simulink model "SH_model3"  (R2022b)
settings: Solver=VariableStepAuto  StartTime=0.0  StopTime=10  RelTol=1e-3
InitFcn:
  | f = 50;
  | V = 12;
  | L = 2.8*10^(-3);
  | I_lim = 1.7;
  | psi = L*I_lim;
  | step_angle = 1.8;
  | m = 2;
  | p = 360/(2*step_angle*m);
  | Jr = 5.4*10^(-6);
  | Ra = 1.5;
  | Rb = Ra;
  | Mst = 0.022;
  | B = 3*10^(-3);
  | Mn = 0.004;
  | n = 2;
  | k = 2;
  | q = 0.005;
  | STEP = 1;
  | DIR = 1;
  | microsteps = 1;
  | ENABLE = 1;
undefined symbols (not defined in the file): sigbuilder_block
settings Model: Creator=longp  LastModifiedBy=longp

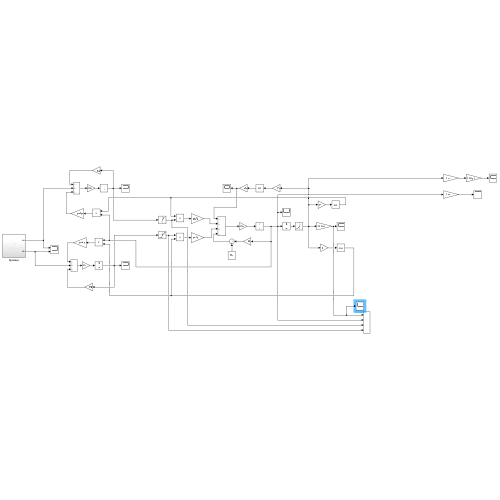
[thumbnail: Simulink's stored preview of the top-level diagram]
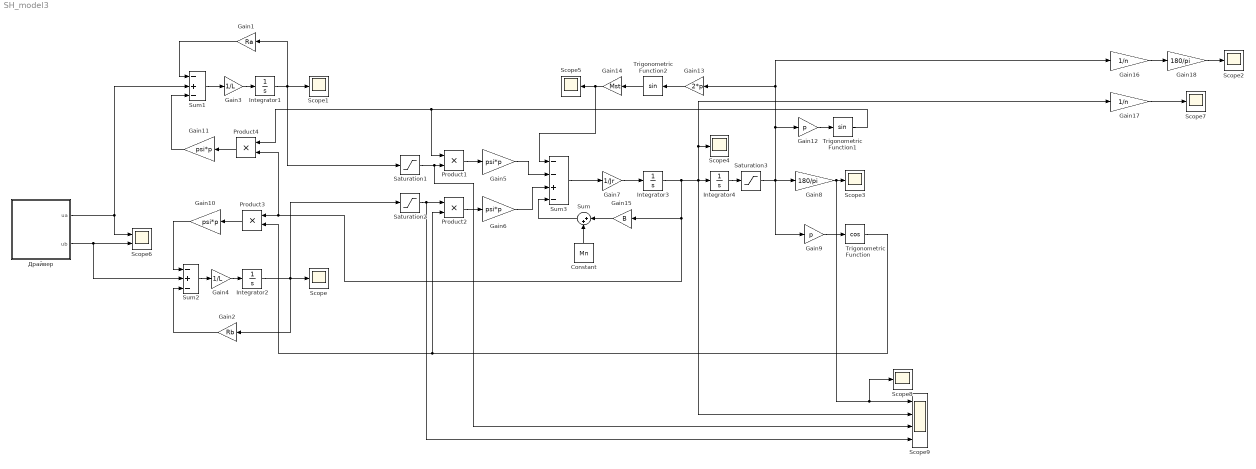
== system SH_model3 ==
  Constant : Constant  Value=Mn
  Gain1 : Gain  Gain=Ra
  Gain{5..6,10..11} (4 alike) : Gain  Gain=psi*p
  Gain12 : Gain  Gain=p
  Gain13 : Gain  Gain=2*p
  Gain14 : Gain  Gain=Mst
  Gain15 : Gain  Gain=B
  Gain16 : Gain  Gain=1/n
  Gain17 : Gain  Gain=1/n
  Gain18 : Gain  Gain=180/pi
  Gain2 : Gain  Gain=Rb
  Gain3 : Gain  Gain=1/L
  Gain4 : Gain  Gain=1/L
  Gain7 : Gain  Gain=1/Jr
  Gain8 : Gain  Gain=180/pi
  Gain9 : Gain  Gain=p
  Integrator{1..4} (4 alike) : Integrator
  Product{1..4} (4 alike) : Product
  Saturation1 : Saturate  UpperLimit=I_lim  LowerLimit=-I_lim
  Saturation2 : Saturate  UpperLimit=I_lim  LowerLimit=-I_lim  ZeroCross=off
  Saturation3 : Saturate  UpperLimit=2*pi  LowerLimit=-2*pi
  Scope{,1..5,7..8} (8 alike) : Scope
  Scope6 : Scope  NumInputPorts=2
  Scope9 : Scope  NumInputPorts=4
  Sum : Sum  Inputs=|++
  Sum1 : Sum  Inputs=-+-
  Sum2 : Sum  Inputs=-+-
  Sum3 : Sum  Inputs=--+-
  Trigonometric Function : Trigonometry  Operator=cos
  Trigonometric Function1 : Trigonometry
  Trigonometric Function2 : Trigonometry
  Драйвер : Subsystem
  wires:
  Integrator1/1 -> Saturation1/1, Gain1/1, Scope1/1
  Gain1/1 -> Sum1/1
  Sum1/1 -> Gain3/1
  Sum2/1 -> Gain4/1
  Integrator2/1 -> Saturation2/1, Gain2/1, Scope/1
  Gain3/1 -> Integrator1/1
  Gain2/1 -> Sum2/3
  Gain4/1 -> Integrator2/1
  Saturation1/1 -> Scope9/3, Product1/2
  Saturation2/1 -> Scope9/4, Product2/1
  Product1/1 -> Gain5/1
  Product2/1 -> Gain6/1
  Gain5/1 -> Sum3/2
  Gain6/1 -> Sum3/3
  Gain7/1 -> Integrator3/1
  Sum3/1 -> Gain7/1
  Integrator4/1 -> Saturation3/1
  Gain9/1 -> Trigonometric Function/1
  Product3/1 -> Gain10/1
  Gain10/1 -> Sum2/1
  Trigonometric Function/1 -> Product2/2, Product3/2
  Product4/1 -> Gain11/1
  Gain11/1 -> Sum1/3
  Gain12/1 -> Trigonometric Function1/1
  Trigonometric Function1/1 -> Product1/1, Product4/1
  Gain13/1 -> Trigonometric Function2/1
  Trigonometric Function2/1 -> Gain14/1
  Gain14/1 -> Sum3/1, Scope5/1
  Integrator3/1 -> Scope9/2, Gain17/1, Scope4/1, Integrator4/1, Product4/2, Product3/1, Gain15/1
  Драйвер/2(ub) -> Sum2/2, Scope6/2
  Драйвер/1(ua) -> Sum1/2, Scope6/1
  Gain8/1 -> Scope8/1, Scope9/1, Scope3/1
  Saturation3/1 -> Gain16/1, Gain13/1, Gain12/1, Gain9/1, Gain8/1
  Constant/1 -> Sum/2
  Gain15/1 -> Sum/1
  Sum/1 -> Sum3/4
  Gain16/1 -> Gain18/1
  Gain17/1 -> Scope7/1
  Gain18/1 -> Scope2/1

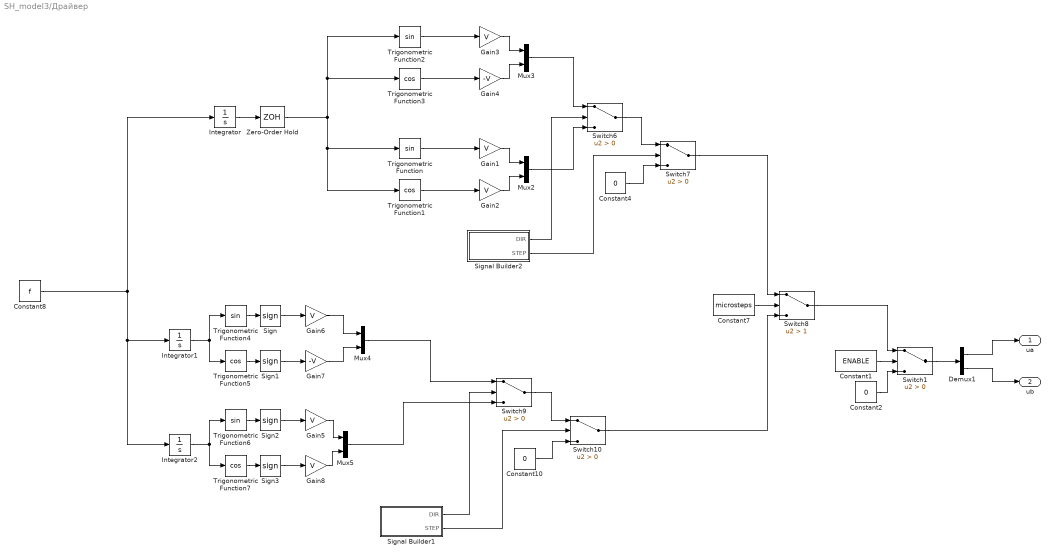
== system SH_model3/Драйвер ==
  Constant1 : Constant  Value=ENABLE
  Constant10 : Constant  Value=0
  Constant2 : Constant  Value=0
  Constant4 : Constant  Value=0
  Constant7 : Constant  Value=microsteps
  Constant8 : Constant  Value=f
  Demux1 : Demux  Outputs=2
  Gain{1..3,5..6,8} (6 alike) : Gain  Gain=V
  Gain4 : Gain  Gain=-V
  Gain7 : Gain  Gain=-V
  Integrator : Integrator
  Integrator1 : Integrator
  Integrator2 : Integrator
  Mux{2..5} (4 alike) : Mux  Inputs=2
  Sign{,1..3} (4 alike) : Signum
  Signal Builder1 : Subsystem  Tag=STV Subsys  LoadFcn=sigbuilder_block('load');  StartFcn=sigbuilder_block('start');  StopFcn=sigbuilder_block('stop');  ClipboardFcn=sigbuilder_block('clipboard');  mask(Sigbuilder block){tuvar=[0:10]}
      mask help: Simulink:masks:SigbuilderBlock_MD
      mask init:
      | if ~strcmp(get_param(bdroot(gcbh),'SimulationStatus'),'stopped') tuvar = sigbuilder_block('maskInit'); end
      settings: CopyFcn=sigbuilder_block('copy');  DeleteFcn=sigbuilder_block('delete');  ModelCloseFcn=sigbuilder_block('modelClose');  PreSaveFcn=sigbuilder_block('preSave');  PauseFcn=sigbuilder_block('pause');  ContinueFcn=sigbuilder_block('continue');  NameChangeFcn=sigbuilder_block('namechange');  OpenFcn=sigbuilder_block('open',[437.6 199.2 550.4 400 ]);  CloseFcn=sigbuilder_block('close');
      mask Display: plot(0, 0, 100, 100,[2, 2, 32, 32, 2], [68, 8, 8, 68, 68],[32, 2], [38, 38], [32, 19, 2],[53, 60, 44], [32, 17, 17, 2],[16, 16, 31, 31]);txt = getActiveGroup(gcbh);text(2, 100, txt,'verticalAlignment', 'top');
  Signal Builder2 : Subsystem  Tag=STV Subsys  LoadFcn=sigbuilder_block('load');  StartFcn=sigbuilder_block('start');  StopFcn=sigbuilder_block('stop');  ClipboardFcn=sigbuilder_block('clipboard');  mask(Sigbuilder block){tuvar=[0:10]}
      mask help: Simulink:masks:SigbuilderBlock_MD
      mask init:
      | if ~strcmp(get_param(bdroot(gcbh),'SimulationStatus'),'stopped') tuvar = sigbuilder_block('maskInit'); end
      settings: CopyFcn=sigbuilder_block('copy');  DeleteFcn=sigbuilder_block('delete');  ModelCloseFcn=sigbuilder_block('modelClose');  PreSaveFcn=sigbuilder_block('preSave');  PauseFcn=sigbuilder_block('pause');  ContinueFcn=sigbuilder_block('continue');  NameChangeFcn=sigbuilder_block('namechange');  OpenFcn=sigbuilder_block('open',[437.6 199.2 550.4 400 ]);  CloseFcn=sigbuilder_block('close');
      mask Display: plot(0, 0, 100, 100,[2, 2, 32, 32, 2], [68, 8, 8, 68, 68],[32, 2], [38, 38], [32, 19, 2],[53, 60, 44], [32, 17, 17, 2],[16, 16, 31, 31]);txt = getActiveGroup(gcbh);text(2, 100, txt,'verticalAlignment', 'top');
  Switch{1,6..7,9..10} (5 alike) : Switch  Criteria=u2 > Threshold  SaturateOnIntegerOverflow=off  InputSameDT=off
  Switch8 : Switch  Criteria=u2 > Threshold  Threshold=1  SaturateOnIntegerOverflow=off  InputSameDT=off
  Trigonometric Function{,2,4,6} (4 alike) : Trigonometry
  Trigonometric Function{1,3,5,7} (4 alike) : Trigonometry  Operator=cos
  Zero-Order Hold : ZeroOrderHold  SampleTime=(2*pi/f)/(2*microsteps)
  ua : Outport
  ub : Outport  Port=2
  wires:
  Switch6/1 -> Switch7/1
  Constant4/1 -> Switch7/3
  Gain2/1 -> Mux2/2
  Gain1/1 -> Mux2/1
  Mux2/1 -> Switch6/3
  Gain4/1 -> Mux3/2
  Gain3/1 -> Mux3/1
  Mux3/1 -> Switch6/1
  Signal Builder2/2(STEP) -> Switch7/2
  Signal Builder2/1(DIR) -> Switch6/2
  Trigonometric Function2/1 -> Gain3/1
  Trigonometric Function3/1 -> Gain4/1
  Trigonometric Function/1 -> Gain1/1
  Trigonometric Function1/1 -> Gain2/1
  Integrator/1 -> Zero-Order Hold/1
  Zero-Order Hold/1 -> Trigonometric Function1/1, Trigonometric Function/1, Trigonometric Function3/1, Trigonometric Function2/1
  Constant7/1 -> Switch8/2
  Integrator1/1 -> Trigonometric Function5/1, Trigonometric Function4/1
  Trigonometric Function4/1 -> Sign/1
  Sign1/1 -> Gain7/1
  Sign/1 -> Gain6/1
  Trigonometric Function5/1 -> Sign1/1
  Gain6/1 -> Mux4/1
  Gain5/1 -> Mux5/1
  Sign3/1 -> Gain8/1
  Integrator2/1 -> Trigonometric Function7/1, Trigonometric Function6/1
  Trigonometric Function6/1 -> Sign2/1
  Trigonometric Function7/1 -> Sign3/1
  Sign2/1 -> Gain5/1
  Gain7/1 -> Mux4/2
  Gain8/1 -> Mux5/2
  Signal Builder1/1(DIR) -> Switch9/2
  Signal Builder1/2(STEP) -> Switch10/2
  Constant10/1 -> Switch10/3
  Switch9/1 -> Switch10/1
  Mux4/1 -> Switch9/1
  Mux5/1 -> Switch9/3
  Switch7/1 -> Switch8/1
  Switch10/1 -> Switch8/3
  Switch1/1 -> Demux1/1
  Demux1/1 -> ua/1
  Demux1/2 -> ub/1
  Constant1/1 -> Switch1/2
  Switch8/1 -> Switch1/1
  Constant2/1 -> Switch1/3
  Constant8/1 -> Integrator/1, Integrator2/1, Integrator1/1

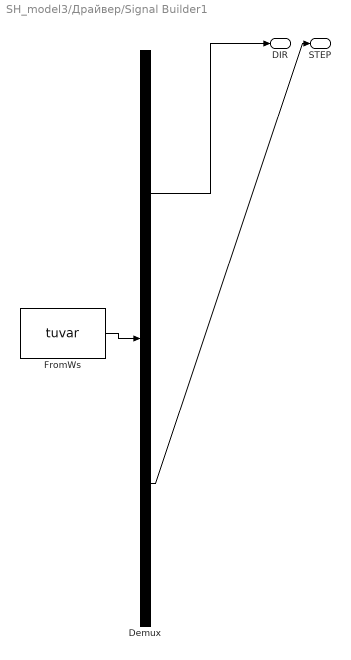
== system SH_model3/Драйвер/Signal Builder1 ==
  Demux : Demux  Tag=STV Demux  Outputs=2
      settings: DisplayOption=none
  FromWs : FromWorkspace  Tag=STV FromWs  VariableName=tuvar
      SigBuilderData=|
      | common.afterFinalStr = 'Extrapolate'
      | common.sampleTime = 0
      | dataSet.timeRange = [0 10]
      | dataSet.name = 'Group 1'
      | sbobj.Groups.Name = 'Group 1'
      | sbobj.Groups.Signals(1).Name = 'DIR'
      | sbobj.Groups.Signals(1).XData = [0 6.4 6.4 10]
      | sbobj.Groups.Signals(1).YData = [1 1 0 0]
      | sbobj.Groups.Signals(2).Name = 'STEP'
      | sbobj.Groups.Signals(2).XData = [0 6.4 6.4 10]
      | sbobj.Groups.Signals(2).YData = [1 1 0 0]
  DIR : Outport  Tag=STV Outport
  STEP : Outport  Tag=STV Outport  Port=2
  wires:
  FromWs/1 -> Demux/1
  Demux/1 -> DIR/1
  Demux/2 -> STEP/1

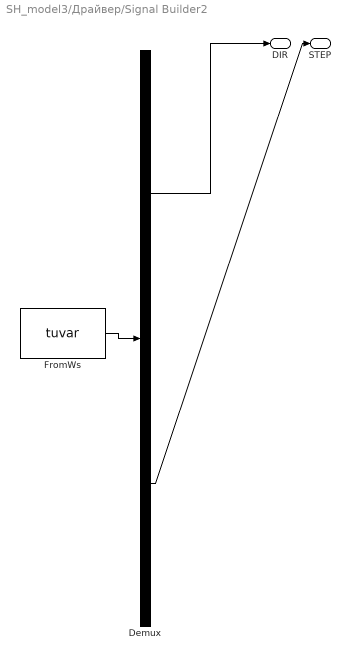
== system SH_model3/Драйвер/Signal Builder2 ==
  Demux : Demux  Tag=STV Demux  Outputs=2
      settings: DisplayOption=none
  FromWs : FromWorkspace  Tag=STV FromWs  VariableName=tuvar
      SigBuilderData=|
      | common.afterFinalStr = 'Extrapolate'
      | common.sampleTime = 0
      | dataSet.timeRange = [0 10]
      | dataSet.name = 'Group 1'
      | sbobj.Groups.Name = 'Group 1'
      | sbobj.Groups.Signals(1).Name = 'DIR'
      | sbobj.Groups.Signals(1).XData = [0 6.4 6.4 10]
      | sbobj.Groups.Signals(1).YData = [1 1 0 0]
      | sbobj.Groups.Signals(2).Name = 'STEP'
      | sbobj.Groups.Signals(2).XData = [0 6.4 6.4 10]
      | sbobj.Groups.Signals(2).YData = [1 1 0 0]
  DIR : Outport  Tag=STV Outport
  STEP : Outport  Tag=STV Outport  Port=2
  wires:
  FromWs/1 -> Demux/1
  Demux/1 -> DIR/1
  Demux/2 -> STEP/1
